simulink model "ask"  (Simulink 5.0)
settings: Solver=ode45  StartTime=0.0  StopTime=10.0  RelTol=1e-3
libraries: commrandsrc2 x1
settings Model: LastModifiedBy=Invitado

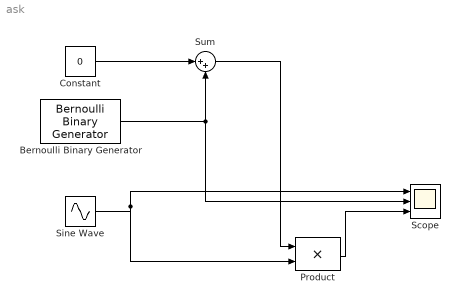
== system ask ==
  Bernoulli Binary Generator : commrandsrc2/Bernoulli Binary Generator  P=0.5  seed=61  Ts=1  frameBased=off  sampPerFrame=1  orient=off
  Constant : Constant  Value=0
  Product : Product  SaturateOnIntegerOverflow=on
  Scope : Scope  NumInputPorts=3
      settings: TimeRange=10  YMin=-2~0~-6  YMax=2~2~6  SampleTime=0.01
  Sine Wave : Sin  Amplitude=2  Frequency=30  SampleTime=0.01
  Sum : Sum  Inputs=|++  SaturateOnIntegerOverflow=on
  wires:
  Constant/1 -> Sum/1
  Sine Wave/1 -> Product/2, Scope/1
  Sum/1 -> Product/1
  Product/1 -> Scope/3
  Bernoulli Binary Generator/1 -> Sum/2, Scope/2
